simulink model "nelinearni_model_njihala"  (R2023a)
settings: Solver=FixedStepAuto  StartTime=0.0  StopTime=15  FixedStep=0.001  MaxStep=0.01  RelTol=1e-3
values from neighbouring files (symbols this model uses):
  b1 = 8.3336*10^(-5)    (= 8.3336e-05)    [Copy_of_CustomPendulumEnvTraining.m]    (also in CustomPendulumEnv.m; CustomPendulumEnvTraining.m; koeficijenti.m; rl_training.m)
  b2 = 2.5*10^(-4)    (= 0.00025)    [Copy_of_CustomPendulumEnvTraining.m]    (also in CustomPendulumEnv.m; CustomPendulumEnvTraining.m; koeficijenti.m; rl_training.m)
  ce = 0.02559    [Copy_of_CustomPendulumEnvTraining.m]    (also in CustomPendulumEnv.m; CustomPendulumEnvTraining.m; koeficijenti.m; rl_training.m)
  cm = 0.02559    [Copy_of_CustomPendulumEnvTraining.m]    (also in CustomPendulumEnv.m; CustomPendulumEnvTraining.m; koeficijenti.m; rl_training.m)
  g = 9.81    [Copy_of_CustomPendulumEnvTraining.m]    (also in CustomPendulumEnv.m; CustomPendulumEnvTraining.m; koeficijenti.m; rl_training.m)
  J0_kapa = 5.5351*10^(-4)    (= 0.00055351)    [Copy_of_CustomPendulumEnvTraining.m]    (also in CustomPendulumEnv.m; CustomPendulumEnvTraining.m; koeficijenti.m; rl_training.m)
  J2_kapa = 3.8533*10^(-4)    (= 0.00038533)    [Copy_of_CustomPendulumEnvTraining.m]    (also in CustomPendulumEnv.m; CustomPendulumEnvTraining.m; koeficijenti.m; rl_training.m)
  L1 = 10.85*10^(-2)    (= 0.1085)    [Copy_of_CustomPendulumEnvTraining.m]    (also in CustomPendulumEnv.m; CustomPendulumEnvTraining.m; koeficijenti.m; rl_training.m)
  l2 = 13.8*10^(-2)    (= 0.138)    [Copy_of_CustomPendulumEnvTraining.m]    (also in CustomPendulumEnv.m; CustomPendulumEnvTraining.m; koeficijenti.m; rl_training.m)
  m2 = 18.1*10^(-3)    (= 0.0181)    [Copy_of_CustomPendulumEnvTraining.m]    (also in CustomPendulumEnv.m; CustomPendulumEnvTraining.m; koeficijenti.m; rl_training.m)
  n = 3.9    [Copy_of_CustomPendulumEnvTraining.m]    (also in CustomPendulumEnv.m; CustomPendulumEnvTraining.m; koeficijenti.m; rl_training.m)
  Ra = 2.19    [Copy_of_CustomPendulumEnvTraining.m]    (also in CustomPendulumEnv.m; CustomPendulumEnvTraining.m; koeficijenti.m; rl_training.m)
settings Model: Creator=Luka  LastModifiedBy=vedran
settings OptimizationCC: ReuseModelBlockBuffer=off
settings HardwareCC: ProdBitPerLong=64  ProdHWDeviceType=Intel->x86-64 (Linux 64)
settings ModelReferenceCC: EnableRefExpFcnMdlSchedulingChecks=on
settings RTWCC: Description=Simulink Desktop Real-Time  SystemTargetFile=sldrt.tlc  TemplateMakefile=sldrt.tmf  RTWCompilerOptimization=on
settings CodeAppCC: MaxIdLength=95
settings SimulinkDesktopRealTimeCC: TargetLibSuffix=_sldrt.a  TargetPreCompLibLocation=C:\Program Files\MATLAB\R2022b\toolbox\sldrt\lib\win64

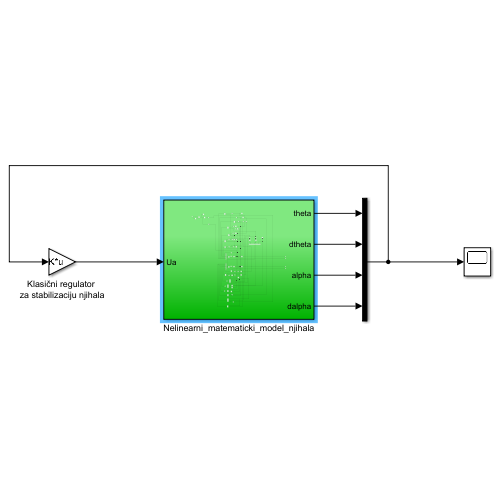
[thumbnail: Simulink's stored preview of the top-level diagram]
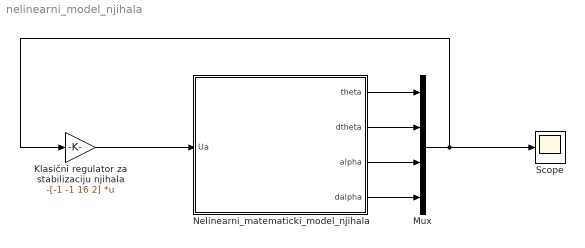
== system nelinearni_model_njihala ==
  Klasični regulator za stabilizaciju njihala : Gain  Gain=-[-1 -1 16 2]  Multiplication=Matrix(K*u)
  Mux : Mux
  Nelinearni_matematicki_model_njihala : Subsystem
  Scope : Scope
  wires:
  Klasični regulator za stabilizaciju njihala/1 -> Nelinearni_matematicki_model_njihala/1(Ua)
  Nelinearni_matematicki_model_njihala/1(theta) -> Mux/1
  Nelinearni_matematicki_model_njihala/2(dtheta) -> Mux/2
  Nelinearni_matematicki_model_njihala/3(alpha) -> Mux/3
  Nelinearni_matematicki_model_njihala/4(dalpha) -> Mux/4
  Mux/1 -> Scope/1, Klasični regulator za stabilizaciju njihala/1

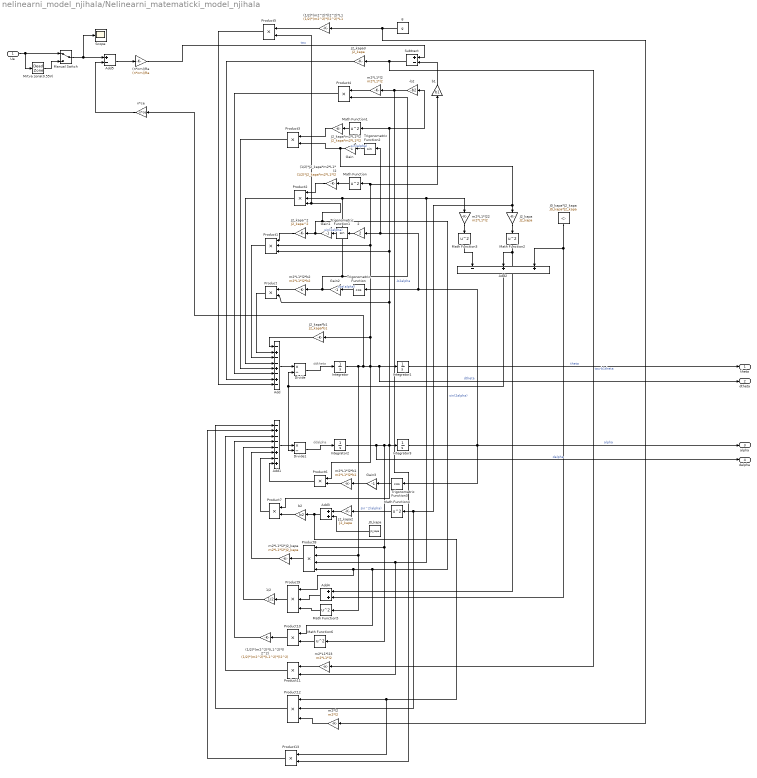
== system nelinearni_model_njihala/Nelinearni_matematicki_model_njihala ==
  note: ddtheta
  note: ddalpha
  Ua : Inport
  (1/2)*(m2^2)*(L1^2)*(l2^2) : Gain  Gain=(1/2)*(m2^2)*(L1^2)*(l2^2)
  (1/2)*(m2^2)*(l2^2)*L1 : Gain  Gain=(1/2)*(m2^2)*(l2^2)*L1
  (1/2)*J2_kapa*m2*L1*l2 : Gain  Gain=(1/2)*J2_kapa*m2*L1*l2
  (n*cm)/Ra : Gain  Gain=(n*cm)/Ra
  -b2 : Gain  Gain=-b2
  1/2 : Gain  Gain=1/2
  2 : Gain  Gain=2
  Add : Sum  Inputs=-+--+-+-
  Add1 : Sum  Inputs=-+---+-+
  Add2 : Sum  Inputs=-++
  Add3 : Sum
  Add4 : Sum
  Add5 : Sum  Inputs=+-
  Divide : Product  Inputs=*/
  Divide1 : Product  Inputs=*/
  Gain{,1..3} (4 alike) : Gain  Gain=-1
  Integrator : Integrator
  Integrator1 : Integrator
  Integrator2 : Integrator
  Integrator3 : Integrator  InitialCondition=pi/16
  J0_kapa : Constant  Value=J0_kapa
  J0_kapa*J2_kapa : Constant  Value=J0_kapa*J2_kapa
  J2_kapa : Gain  Gain=J2_kapa
  J2_kapa*b1 : Gain  Gain=J2_kapa*b1
  J2_kapa*m2*L1*l2 : Gain  Gain=J2_kapa*m2*L1*l2
  J2_kapa2 : Gain  Gain=J2_kapa
  J2_kapa3 : Gain  Gain=J2_kapa
  J2_kapa^2 : Gain  Gain=J2_kapa^2
  Manual Switch : ManualSwitch
  Math Function{,1..6} (7 alike) : Math  Operator=square
  Mrtva zona(0.55V) : DeadZone  LowerValue=-0.55  UpperValue=0.55
  Product{,3..7,10..11,13} (9 alike) : Product
  Product{1..2,9,12} (4 alike) : Product  Inputs=3
  Product8 : Product  Inputs=4
  Scope : Scope
  Subtract : Sum  Inputs=+-
  Trigonometric Function : Trigonometry  Operator=cos
  Trigonometric Function1 : Trigonometry
  Trigonometric Function2 : Trigonometry
  Trigonometric Function3 : Trigonometry  Operator=cos
  b1 : Gain  Gain=b1
  b2 : Gain  Gain=b2
  g : Constant  Value=g
  m2*L1*l2 : Gain  Gain=m2*L1*l2
  m2*L1*l2*J2_kapa : Gain  Gain=m2*L1*l2*J2_kapa
  m2*L1*l2*b1 : Gain  Gain=m2*L1*l2*b1
  m2*L1*l2*b2 : Gain  Gain=m2*L1*l2*b2
  m2*L1*l22 : Gain  Gain=m2*L1*l2
  m2*L1*l23 : Gain  Gain=m2*L1*l2
  m2*l2 : Gain  Gain=m2*l2
  n*ce : Gain  Gain=n*ce
  theta : Outport
  dtheta : Outport  Port=2
  alpha : Outport  Port=3
  dalpha : Outport  Port=4
  wires:
  Add4/1 -> Product9/2
  Add3/1 -> Product13/1, Product12/1, b2/1
  Trigonometric Function2/1 -> Gain/1  "sin(alpha)"
  Product3/1 -> Add/5
  m2*L1*l2*J2_kapa/1 -> Add1/6
  Add1/1 -> Divide1/1
  m2*L1*l2/1 -> Product4/1
  Add2/1 -> Divide1/2, Divide/2
  Trigonometric Function/1 -> Gain2/1  "cos(alpha)"
  m2*L1*l2*b2/1 -> Product/1
  Integrator/1 -> Math Function5/1, Product8/2, n*ce/1, Product6/1, b1/1, Math Function/1, Product1/2, J2_kapa*b1/1, dtheta/1, Integrator1/1  "dtheta"
  Math Function3/1 -> Add2/1
  Product10/1 -> (1/2)*(m2^2)*(L1^2)*(l2^2)/1
  Divide1/1 -> Integrator2/1
  m2*l2/1 -> Product12/3
  Integrator2/1 -> dalpha/1, Math Function6/1, Product8/1, Product7/1, -b2/1, Math Function1/1, Product1/3, Product/2, Integrator3/1  "dalpha"
  J2_kapa*b1/1 -> Add/1
  m2*L1*l2*b1/1 -> Product6/2
  2/1 -> Trigonometric Function1/1
  Gain1/1 -> J2_kapa^2/1, Product10/1, Product9/1, Product8/4, Product5/2, Product2/3  "sin(2alpha)"
  J2_kapa3/1 -> Add/7
  J2_kapa^2/1 -> Product1/1
  Product1/1 -> Add/3
  (1/2)*(m2^2)*(L1^2)*(l2^2)/1 -> Add1/4
  Product5/1 -> Add/8
  Math Function1/1 -> J2_kapa*m2*L1*l2/1
  (1/2)*(m2^2)*(l2^2)*L1/1 -> Product5/1
  m2*L1*l23/1 -> Product11/1
  Product/1 -> Add/2
  J0_kapa/1 -> Add3/2
  J0_kapa*J2_kapa/1 -> Add4/2, Add2/3
  Product4/1 -> Add/6
  Add/1 -> Divide/1
  J2_kapa2/1 -> Add3/1
  Product7/1 -> Add1/7
  g/1 -> (1/2)*(m2^2)*(l2^2)*L1/1, m2*l2/1
  Math Function4/1 -> J2_kapa2/1  "sin^2(alpha)"
  J2_kapa/1 -> Math Function2/1
  Divide/1 -> Integrator/1
  m2*L1*l22/1 -> Math Function3/1
  Math Function/1 -> (1/2)*J2_kapa*m2*L1*l2/1
  1/2/1 -> Add1/5
  Product2/1 -> Add/4
  Math Function2/1 -> Add4/1, Add2/2
  (1/2)*J2_kapa*m2*L1*l2/1 -> Product2/1
  Product12/1 -> Add1/1
  Product8/1 -> m2*L1*l2*J2_kapa/1
  Integrator1/1 -> theta/1  "theta"
  Product6/1 -> Add1/8
  Product9/1 -> 1/2/1
  Math Function5/1 -> Product9/3
  Product11/1 -> Add1/3
  (n*cm)/Ra/1 -> Subtract/1  "tau"
  Math Function6/1 -> Product10/2
  J2_kapa*m2*L1*l2/1 -> Product3/1
  -b2/1 -> Product13/2, m2*L1*l2/1  "-b2alpha"
  Trigonometric Function3/1 -> Gain3/1
  b2/1 -> Product7/2
  n*ce/1 -> Add5/2
  Add5/1 -> (n*cm)/Ra/1
  Ua/1 -> Mrtva zona(0.55V)/1, Manual Switch/1
  b1/1 -> Subtract/2
  Subtract/1 -> J2_kapa3/1, m2*L1*l23/1  "tau-b1theta"
  Product13/1 -> Add1/2
  Gain/1 -> Product12/2, Math Function4/1, J2_kapa/1, Product3/2
  Trigonometric Function1/1 -> Gain1/1  "sin(2alpha)"
  Gain2/1 -> m2*L1*l2*b2/1, Product4/2, Product11/2, Product8/3, m2*L1*l22/1, Product2/2
  Gain3/1 -> m2*L1*l2*b1/1
  Manual Switch/1 -> Scope/1, Add5/1
  Mrtva zona(0.55V)/1 -> Manual Switch/2
  Integrator3/1 -> Trigonometric Function2/1, 2/1, Trigonometric Function/1, alpha/1, Trigonometric Function3/1  "alpha"
